simulink model "Simulink_Simulation"  (Simulink 10.1)
settings: Solver=ode23t  StartTime=0.0  StopTime=0.08  RelTol=1e-3  EnableMultiTasking=on
libraries: powerlib x13, powerlib_meascontrol x4
settings Model: Creator=asus1  LastModifiedBy=x64
settings DataIOCC: LimitDataPoints=on
settings DebuggingCC: UnderspecifiedInitializationDetection=Simplified  MergeDetectMultiDrivingBlocksExec=error  SolverPrmCheckMsg=warning
settings GRTTargetCC: CombineOutputUpdateFcns=on  GRTInterface=off
settings ConfigComp: CovSFcnEnable=off
settings SimscapeCC: SimscapeNormalizeSystem=off

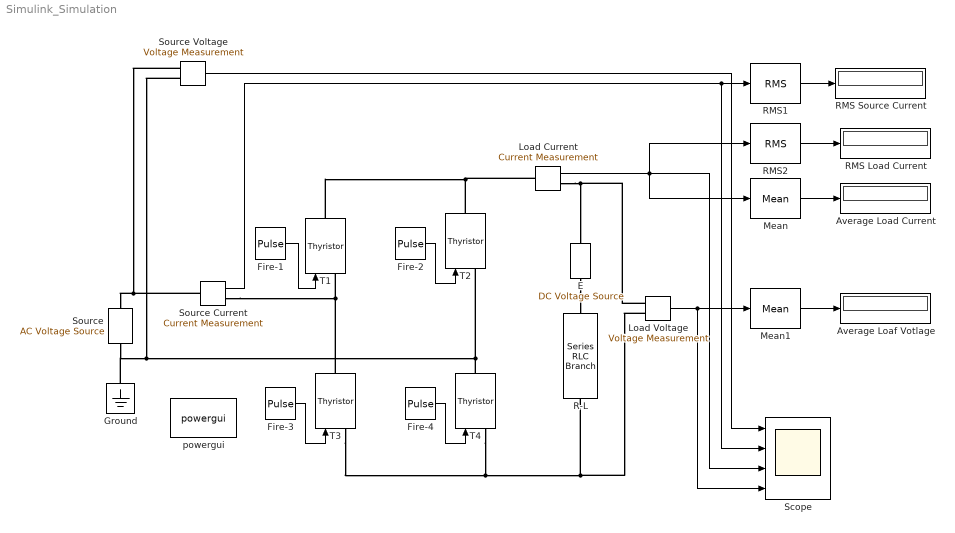
== system Simulink_Simulation ==
  Average Load Current : Display
  Average Loaf Votlage : Display
  E : powerlib/Electrical Sources/DC Voltage Source  Amplitude=220  Measurements=None
  "Fire-1 " : DiscretePulseGenerator  PulseType=Time based  Amplitude=5  Period=0.02  PulseWidth=5  PhaseDelay=90*0.02/360  VectorParams1D=off
  Fire-2 : DiscretePulseGenerator  PulseType=Time based  Amplitude=5  Period=0.02  PulseWidth=5  PhaseDelay=270*0.02/360  VectorParams1D=off
  Fire-3 : DiscretePulseGenerator  PulseType=Time based  Amplitude=5  Period=0.02  PulseWidth=5  PhaseDelay=270*0.02/360  VectorParams1D=off
  Fire-4 : DiscretePulseGenerator  PulseType=Time based  Amplitude=5  Period=0.02  PulseWidth=5  PhaseDelay=90*0.02/360  VectorParams1D=off
  Ground : powerlib/Elements/Ground  LConnTagsString=a
  Load Current : powerlib/Measurements/Current Measurement  PhasorSimulation=off  OutputType=Complex  PSBequivalent=0
  "Load Voltage " : powerlib/Measurements/Voltage Measurement  PhasorSimulation=off  OutputType=Complex  PSBequivalent=0
  Mean : powerlib_meascontrol/Measurements/Mean  Freq=50  Vinit=0  Ts=0
  Mean1 : powerlib_meascontrol/Measurements/Mean  Freq=50  Vinit=0  Ts=0
  R-L : powerlib/Elements/Series RLC Branch  LConnTagsString=__new0  RConnTagsString=__new0  BranchType=RL  Resistance=1  Inductance=1e-2  SetiL0=off  InitialCurrent=0  Capacitance=1e-6  Setx0=off  InitialVoltage=0  Measurements=None
  RMS Load Current : Display
  RMS Source Current : Display
  RMS1 : powerlib_meascontrol/Measurements/RMS  TrueRMS=on  Freq=50  RMSInit=0  Ts=0
  RMS2 : powerlib_meascontrol/Measurements/RMS  TrueRMS=on  Freq=50  RMSInit=0  Ts=0
  Scope : Scope  NumInputPorts=4
  Source : powerlib/Electrical Sources/AC Voltage Source  Amplitude=220*sqrt(2)  Phase=0  Frequency=50  SampleTime=0  Measurements=None  BusType=swing  Pref=10e3  Qref=0  Qmin=-inf  Qmax=+inf
  "Source Current " : powerlib/Measurements/Current Measurement  PhasorSimulation=off  OutputType=Complex  PSBequivalent=0
  Source Voltage : powerlib/Measurements/Voltage Measurement  PhasorSimulation=off  OutputType=Complex  PSBequivalent=0
  T1 : powerlib/Power Electronics/Thyristor  Ron=0.001  Lon=0  Vf=0.001  IC=0  Rs=5000  Cs=250e-2  Measurements=off
  T2 : powerlib/Power Electronics/Thyristor  Ron=0.001  Lon=0  Vf=0.001  IC=0  Rs=5000  Cs=250e-2  Measurements=off
  T3 : powerlib/Power Electronics/Thyristor  Ron=0.001  Lon=0  Vf=0.01  IC=0  Rs=5000  Cs=250e-2  Measurements=off
  T4 : powerlib/Power Electronics/Thyristor  Ron=0.001  Lon=0  Vf=0.001  IC=0  Rs=5000  Cs=250e-2  Measurements=off
  powergui : powerlib/powergui  Priority=1  SimulationMode=Discrete  SampleTime=1e-6  frequency=60  Iterations=50  frequencyindice=50  Pbase=100e6  ErrMax=1e-4  UnitsV=kV  UnitsW=MW  buscounter=0  FunctionMessages=off  echomessages=off  EnableUseOfTLC=off  CurrentSourceSwitches=off  DisableSnubberDevices=off  DisableRonSwitches=off  DisableVfSwitches=off  DisplayEquations=off  AutomaticDiscreteSolvers=off  SolverType=Tustin  Interpol=off  ExternalGateDelay=off  methode=off  Ts=100  x0status=blocks  SPID=off  SwTol=0  HookPort=off  NonlinearTolerance=1e-4  nMaxIteration=100  ContinueOnMaxIteration=off  RestoreLinks=warning  ResistiveCurrentMeasurement=off  Frange=[0:2:500]  Ylog=off  Xlog=on  ShowGrid=off  save=off  variable=ZData  structure=0  ZoomFFT=off  StartTime=0.0  cycles=1  DisplayStyle=1  fundamental=60  FreqAxis=off  MaxFrequency=1000  frequencyindicesteady=1  RmsSteady=1  display=off
  wires:
  "Fire-1 "/1 -> T1/1
  Fire-2/1 -> T2/1
  Fire-3/1 -> T3/1
  Fire-4/1 -> T4/1
  "Source Current "/1 -> Scope/2, RMS1/1
  RMS1/1 -> RMS Source Current/1
  Load Current/1 -> Scope/3, Mean/1, RMS2/1
  RMS2/1 -> RMS Load Current/1
  Mean/1 -> Average Load Current/1
  Mean1/1 -> Average Loaf Votlage/1
  "Load Voltage "/1 -> Scope/4, Mean1/1
  Source Voltage/1 -> Scope/1
  connections:
  T3/RConn1 -- "Source Current "/RConn1 -- T1/LConn1
  T4/RConn1 -- Ground/LConn1 -- Source/LConn1 -- Source Voltage/LConn2 -- T2/LConn1
  E/LConn1 -- R-L/LConn1
  T1/RConn1 -- Load Current/LConn1 -- T2/RConn1
  T3/LConn1 -- T4/LConn1 -- R-L/RConn1 -- "Load Voltage "/LConn2
  "Source Current "/LConn1 -- Source Voltage/LConn1 -- Source/RConn1
  Load Current/RConn1 -- "Load Voltage "/LConn1 -- E/RConn1
